simulink model "Test_Word_Multiplexer_2_to_1"  (R2023a)
settings: Solver=ode45  StartTime=0.0  StopTime=len  RelTol=1e-3  EnableMultiTasking=on
libraries: Miscellaneous x3, simulink x1, Word_Multiplexers_Lib x1
settings Model: Creator=N  LastModifiedBy=Jozko Mrkvicka
settings SolverCC: AlgebraicLoopSolver=TrustRegion
settings DataIOCC: SaveFormat=Array  ReturnWorkspaceOutputs=off
settings OptimizationCC: LifeSpan=inf
settings DebuggingCC: UnconnectedInputMsg=warning  UnconnectedOutputMsg=warning  UnconnectedLineMsg=warning  SFUnexpectedBacktrackingDiag=warning  SFNoUnconditionalDefaultTransitionDiag=warning  ArithmeticOperatorsInVariantConditions=warning
settings HardwareCC: ProdWordSize=32
settings ModelReferenceCC: EnableRefExpFcnMdlSchedulingChecks=on
settings SFSimCC: SimUseLocalCustomCode=off  CustomCodeUndefinedFunction=UseInterfaceOnly
settings RTWCC: RTWUseLocalCustomCode=off
settings CodeAppCC: StateflowObjectComments=on
settings GRTTargetCC: TargetLangStandard=C89/C90 (ANSI)
settings ConfigComp: CovMetricSettings=dw  CovSaveCumulativeToWorkspaceVar=on  CovSaveSingleToWorkspaceVar=on  CovExternalEMLEnable=off

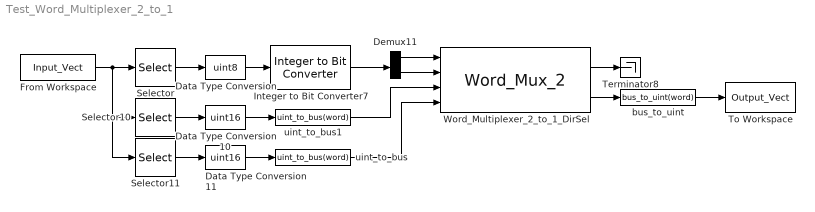
== system Test_Word_Multiplexer_2_to_1 ==
  Data Type Conversion : DataTypeConversion  OutDataTypeStr=uint8  SaturateOnIntegerOverflow=off  RndMeth=Floor
  Data Type Conversion10 : DataTypeConversion  OutDataTypeStr=uint16  SaturateOnIntegerOverflow=off  RndMeth=Floor
  Data Type Conversion11 : DataTypeConversion  OutDataTypeStr=uint16  SaturateOnIntegerOverflow=off  RndMeth=Floor
  Demux11 : Demux  Outputs=2
  From Workspace : FromWorkspace  VariableName=Input_Vect  SampleTime=1  Interpolate=off  ZeroCross=off  OutputAfterFinalValue=Holding final value
  Integer to Bit Converter7 : simulink/Logic and Bit Operations/Integer to Bit Converter  nbits=2  signedInputValues=Unsigned  bitOrder=MSB first  outDtype=boolean
      settings: LibrarySourceBlock=|
      | commutil2/Integer to Bit
      | Converter
  Selector : Selector  IndexMode=Zero-based  InputPortWidth=3  SampleTime=1  IndexOptions=Index vector (dialog)  Indices=0  OutputSizes=1
  Selector10 : Selector  IndexMode=Zero-based  InputPortWidth=3  IndexOptions=Index vector (dialog)  Indices=1  OutputSizes=1
  Selector11 : Selector  IndexMode=Zero-based  InputPortWidth=3  IndexOptions=Index vector (dialog)  Indices=2  OutputSizes=1
  Terminator8 : Terminator
  To Workspace : ToWorkspace  VariableName=Output_Vect  SampleTime=1
  Word_Multiplexer_2_to_1_DirSel : Word_Multiplexers_Lib/Word_Mux_2  SystemSampleTime=-1  VariantActivationTime=update diagram  Latency=0  AutoFrameSizeCalculation=off
  bus_to_uint : Miscellaneous/bus_to_uint(word)
  uint_to_bus : Miscellaneous/uint_to_bus(word)
  uint_to_bus1 : Miscellaneous/uint_to_bus(word)
  wires:
  Word_Multiplexer_2_to_1_DirSel/2 -> bus_to_uint/1
  Integer to Bit Converter7/1 -> Demux11/1
  Selector/1 -> Data Type Conversion/1
  Data Type Conversion/1 -> Integer to Bit Converter7/1
  From Workspace/1 -> Selector11/1, Selector10/1, Selector/1
  Selector10/1 -> Data Type Conversion10/1
  Selector11/1 -> Data Type Conversion11/1
  Data Type Conversion10/1 -> uint_to_bus1/1
  Data Type Conversion11/1 -> uint_to_bus/1
  uint_to_bus1/1 -> Word_Multiplexer_2_to_1_DirSel/3
  uint_to_bus/1 -> Word_Multiplexer_2_to_1_DirSel/4
  bus_to_uint/1 -> To Workspace/1
  Demux11/1 -> Word_Multiplexer_2_to_1_DirSel/1
  Demux11/2 -> Word_Multiplexer_2_to_1_DirSel/2
  Word_Multiplexer_2_to_1_DirSel/1 -> Terminator8/1
